simulink subsystem "pololu_37D_pos_second_order_discrete"  (R2023b)
settings: Solver=VariableStepAuto  StartTime=0.0  StopTime=10.0  RelTol=1e-3
undefined symbols (not defined in the file): sys_dis
settings Model: Creator=kiraa  LastModifiedBy=paoli

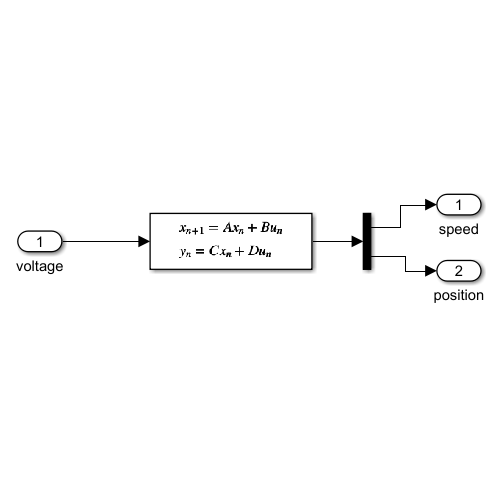
[thumbnail: Simulink's stored preview of the top-level diagram]
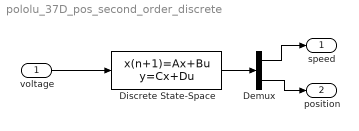
== system pololu_37D_pos_second_order_discrete ==
  voltage : Inport
  Demux : Demux  Outputs=2
  Discrete State-Space : DiscreteStateSpace  A=sys_dis.A  B=sys_dis.B  C=eye(2)  D=[0; 0]  SampleTime=-1
  speed : Outport
  position : Outport  Port=2
  wires:
  voltage/1 -> Discrete State-Space/1
  Demux/1 -> speed/1
  Demux/2 -> position/1
  Discrete State-Space/1 -> Demux/1
